simulink model "online"  (R2014a)
settings: Solver=ode45  StartTime=0.0  StopTime=10.0  RelTol=1e-3
libraries: dsparch4 x5
settings Model: Creator=Josete Flowww  LastModifiedBy=Josete Flowww

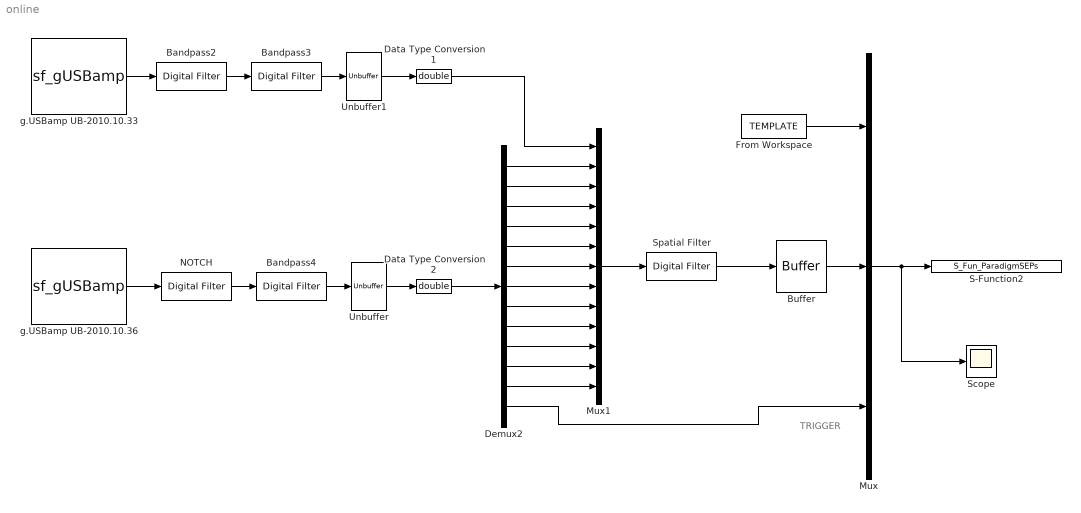
== system online ==
  note: TRIGGER
  Bandpass2 : dsparch4/Digital Filter  TypePopup=IIR (poles & zeros)  IIRFiltStruct=Direct form II transposed  AllPoleFiltStruct=Direct form  FIRFiltStruct=Direct form  CoeffSource=Specify via dialog  NumCoeffs=[1 2]  DenCoeffs=[1 0.1]  BiQuadCoeffs=[1 0.3 0.4 1 0.1 0.2]  LatticeCoeffs=[0.2 0.4]  denIgnore=on  FiltPerSampPopup=One filter per frame  IC=0  ICnum=0  ICden=0  roundingMode=Floor  overflowMode=off  ScaleValues=1  scaleValueFracLength=14  stageInFracLength=15  stageOutFracLength=15  FilterSource=dfilt object  dfiltObjectName=HdNotch  InputProcessing=Inherited (this choice will be removed - see release notes)
  Bandpass3 : dsparch4/Digital Filter  TypePopup=IIR (poles & zeros)  IIRFiltStruct=Direct form II transposed  AllPoleFiltStruct=Direct form  FIRFiltStruct=Direct form  CoeffSource=Specify via dialog  NumCoeffs=[1 2]  DenCoeffs=[1 0.1]  BiQuadCoeffs=[1 0.3 0.4 1 0.1 0.2]  LatticeCoeffs=[0.2 0.4]  denIgnore=on  FiltPerSampPopup=One filter per frame  IC=0  ICnum=0  ICden=0  roundingMode=Floor  overflowMode=off  ScaleValues=1  scaleValueFracLength=14  stageInFracLength=15  stageOutFracLength=15  FilterSource=dfilt object  dfiltObjectName=BP_SEP  InputProcessing=Inherited (this choice will be removed - see release notes)
  Bandpass4 : dsparch4/Digital Filter  TypePopup=IIR (poles & zeros)  IIRFiltStruct=Direct form II transposed  AllPoleFiltStruct=Direct form  FIRFiltStruct=Direct form  CoeffSource=Specify via dialog  NumCoeffs=[1 2]  DenCoeffs=[1 0.1]  BiQuadCoeffs=[1 0.3 0.4 1 0.1 0.2]  LatticeCoeffs=[0.2 0.4]  denIgnore=on  FiltPerSampPopup=One filter per frame  IC=0  ICnum=0  ICden=0  roundingMode=Floor  overflowMode=off  ScaleValues=1  scaleValueFracLength=14  stageInFracLength=15  stageOutFracLength=15  FilterSource=dfilt object  dfiltObjectName=BP_SEP  InputProcessing=Inherited (this choice will be removed - see release notes)
  Buffer : Buffer  TreatMby1Signals=One channel
  Data Type Conversion1 : DataTypeConversion  OutDataTypeStr=double
  Data Type Conversion2 : DataTypeConversion  OutDataTypeStr=double
  Demux2 : Demux  Outputs=13
  From Workspace : FromWorkspace  VariableName=TEMPLATE  SampleTime=1/2400
  Mux : Mux  Inputs=3
  Mux1 : Mux  Inputs=13
  NOTCH : dsparch4/Digital Filter  TypePopup=IIR (poles & zeros)  IIRFiltStruct=Direct form II transposed  AllPoleFiltStruct=Direct form  FIRFiltStruct=Direct form  CoeffSource=Specify via dialog  NumCoeffs=[1 2]  DenCoeffs=[1 0.1]  BiQuadCoeffs=[1 0.3 0.4 1 0.1 0.2]  LatticeCoeffs=[0.2 0.4]  denIgnore=on  FiltPerSampPopup=One filter per frame  IC=0  ICnum=0  ICden=0  roundingMode=Floor  overflowMode=off  ScaleValues=1  scaleValueFracLength=14  stageInFracLength=15  stageOutFracLength=15  FilterSource=dfilt object  dfiltObjectName=HdNotch  InputProcessing=Inherited (this choice will be removed - see release notes)
  S-Function2 : S-Function  FunctionName=S_Fun_ParadigmSEPs  EnableBusSupport=off
  Scope : Scope
  Spatial Filter : dsparch4/Digital Filter  TypePopup=IIR (poles & zeros)  IIRFiltStruct=Direct form II transposed  AllPoleFiltStruct=Direct form  FIRFiltStruct=Direct form  CoeffSource=Specify via dialog  NumCoeffs=[1 2]  DenCoeffs=[1 0.1]  BiQuadCoeffs=[1 0.3 0.4 1 0.1 0.2]  LatticeCoeffs=[0.2 0.4]  denIgnore=on  FiltPerSampPopup=One filter per frame  IC=0  ICnum=0  ICden=0  roundingMode=Floor  overflowMode=off  ScaleValues=1  scaleValueFracLength=14  stageInFracLength=15  stageOutFracLength=15  FilterSource=dfilt object  dfiltObjectName=Spatial_SEP  InputProcessing=Inherited (this choice will be removed - see release notes)
  Unbuffer : Unbuffer
  Unbuffer1 : Unbuffer
  g.USBamp UB-2010.10.33 : S-Function  FunctionName=sf_gUSBamp  Parameters=cfg,snr  EnableBusSupport=off  mask{cfg=currentCFG_RecordMEPs_UA-2008.06.26.cfg, snr=UA-2008.06.26}
      mask prompts: cfg "Configuration"; snr "Serial"
      mask help: Enter configuration file and serial
      settings: OpenFcn=|
      | %gua_click
      | gua_block_cfg
      mask Display: image(imread('USB_symb.tif'))
  g.USBamp UB-2010.10.36 : S-Function  FunctionName=sf_gUSBamp  Parameters=cfg,snr  EnableBusSupport=off  mask{cfg=currentCFG_RecordMEPs_UA-2008.06.26.cfg, snr=UA-2008.06.26}
      mask prompts: cfg "Configuration"; snr "Serial"
      mask help: Enter configuration file and serial
      settings: OpenFcn=|
      | %gua_click
      | gua_block_cfg
      mask Display: image(imread('USB_symb.tif'))
  wires:
  Mux/1 -> Scope/1, S-Function2/1
  Bandpass2/1 -> Bandpass3/1
  NOTCH/1 -> Bandpass4/1
  Unbuffer/1 -> Data Type Conversion2/1
  Unbuffer1/1 -> Data Type Conversion1/1
  Bandpass3/1 -> Unbuffer1/1
  Bandpass4/1 -> Unbuffer/1
  g.USBamp UB-2010.10.36/1 -> NOTCH/1
  g.USBamp UB-2010.10.33/1 -> Bandpass2/1
  Data Type Conversion2/1 -> Demux2/1
  Data Type Conversion1/1 -> Mux1/1
  From Workspace/1 -> Mux/1
  Demux2/13 -> Mux/3
  Buffer/1 -> Mux/2
  Demux2/12 -> Mux1/13
  Demux2/11 -> Mux1/12
  Demux2/10 -> Mux1/11
  Demux2/9 -> Mux1/10
  Demux2/8 -> Mux1/9
  Demux2/7 -> Mux1/8
  Demux2/6 -> Mux1/7
  Demux2/5 -> Mux1/6
  Demux2/4 -> Mux1/5
  Demux2/3 -> Mux1/4
  Demux2/2 -> Mux1/3
  Demux2/1 -> Mux1/2
  Mux1/1 -> Spatial Filter/1
  Spatial Filter/1 -> Buffer/1
